simulink model "TestBenchModel"  (R2019b)
settings: Solver=VariableStepAuto  StartTime=0.0  StopTime=60  FixedStep=0.0001  RelTol=1e-3  EnableMultiTasking=on
InitFcn:
  | TestBenchData;
StartFcn:
  | TestBenchData;
values from neighbouring files (symbols this model uses):
  C = 0.0056    [TestBenchData.m]
  C1 = C    (= 0.0056)    [TestBenchData.m]
  C2 = C1    (= 0.0056)    [TestBenchData.m]
  C3 = C1    (= 0.0056)    [TestBenchData.m]
  C4 = C1    (= 0.0056)    [TestBenchData.m]
  C5 = C1    (= 0.0056)    [TestBenchData.m]
  C6 = C1    (= 0.0056)    [TestBenchData.m]
  Cfc = 0.35    [TestBenchData.m]
  Fs = 1000    [TestBenchData.m]
  glg = 4    [TestBenchData.m]
  gug = 3    [TestBenchData.m]
  Ic1 = 0.05*10^(-3)    (= 5e-05)    [TestBenchData.m]
  Ic4 = Ic3    (= 0.00012)    [TestBenchData.m]
  Ic_mf = 1.1420e-04    (= 0.0001142)    [TestBenchData.m]
  Ifc_1 = 0.003*10^(-3)    (= 3e-06)    [TestBenchData.m]
  Ifc_2 = 0.003*10^(-3)    (= 3e-06)    [TestBenchData.m]
  Imotor = 0.00068    [TestBenchData.m]
  Iprop = gml^2*I_ML + I_GL + Iprop0    [TestBenchData.m]
  Kc1 = 41.9*10^3    (= 41900)    [TestBenchData.m]
  Kc2 = Kc1    (= 41900)    [TestBenchData.m]
  Kc3 = 31*10^3    (= 31000)    [TestBenchData.m]
  Kc4 = Kc3    (= 31000)    [TestBenchData.m]
  Kc5 = 138*10^3    (= 138000)    [TestBenchData.m]
  Kc6 = Kc5    (= 138000)    [TestBenchData.m]
  Kc_mf = 1.9039e+05    (= 190390)    [TestBenchData.m]
  Kfc = 90    [TestBenchData.m]
  Klg = 44.3*10^3    (= 44300)    [TestBenchData.m]
  Km1 = 5.4*10^3    (= 5400)    [TestBenchData.m]
  Km2 = 20*10^3    (= 20000)    [TestBenchData.m]
  Kug = 43.3*10^3    (= 43300)    [TestBenchData.m]
  lg = C1    (= 0.0056)    [TestBenchData.m]
  M1 = S1    (= 0.0056)    [TestBenchData.m]
  M2 = M1    (= 0.0056)    [TestBenchData.m]
  n = 3221    [TestBenchData.m]
  n_idle = 0    [TestBenchData.m]
  Nmill = 12    [TestBenchData.m]
  P = 1150    [TestBenchData.m]
  prop_blades = 4    [TestBenchData.m]
  S = 0.0056    [TestBenchData.m]
  S1 = S    (= 0.0056)    [TestBenchData.m]
  S2 = S1    (= 0.0056)    [TestBenchData.m]
  S3 = S1    (= 0.0056)    [TestBenchData.m]
  S4 = S1    (= 0.0056)    [TestBenchData.m]
  S5 = S1    (= 0.0056)    [TestBenchData.m]
  T = P/(n/9.55)    (= 3.40965538653)    [TestBenchData.m]
  Tice = 100000    [TestBenchData.m]
  To = 0.2    [TestBenchData.m]
  Todelta = 0.5    [TestBenchData.m]
  ug = C1    (= 0.0056)    [TestBenchData.m]
  W = 131.9469    [TestBenchData.m]
  x4 = 0.06/4    (= 0.015)    [TestBenchData.m]
  x8 = 0.02/4    (= 0.005)    [TestBenchData.m]
  Z = 4    [TestBenchData.m]
  z1 = 17    [TestBenchData.m]
  z2 = 42    [TestBenchData.m]
undefined symbols (not defined in the file or in its folder): C1_22, C1_3, C_crank, C_cyl, Data, Iem, Is1, Is2, Is3, Is4, Is5, K1_11, K1_13, K1_15, K1_21, K1_23, K1_5, K1_7, K1_9, Ks1, Ks2, Ks3, Ks4, Ks5, Ks_mf, RPM, Tu
libraries: fl_lib x201, nesl_utility x92, simulink x22, dspstat3 x1
(part 2 of 3)

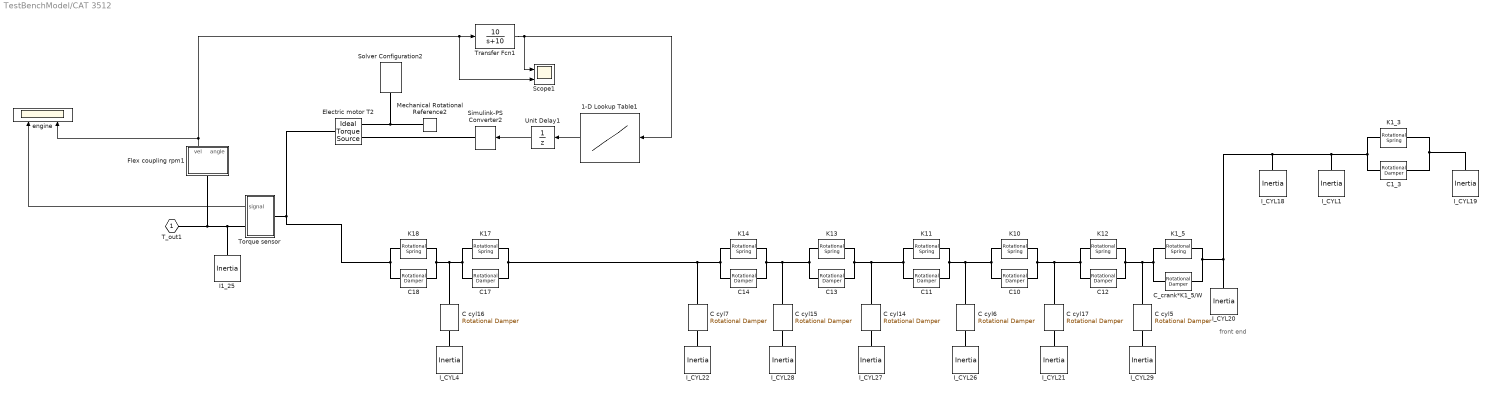
== system TestBenchModel/CAT 3512 ==
  note: front end
  " K1_5" : fl_lib/Mechanical/Rotational Elements/Rotational Spring  spr_rate=K1_5 N*m/rad  w_specify=off  w_priority=None  w=0 rad/s  w_nominal_specify=off  w_nominal_unit=rad/s  w_nominal_value=1  t_specify=off  t_priority=None  t=0 N*m  t_nominal_specify=off  t_nominal_unit=N*m  t_nominal_value=1  phi_specify=on  phi_priority=High  phi=0 rad  phi_nominal_specify=off  phi_nominal_unit=rad  phi_nominal_value=1
      settings: SourceProductName=Simscape
  " engine" : Scope  NumInputPorts=2
  1-D Lookup Table1 : Lookup_n-D  NumberOfTableDimensions=1  BreakpointsForDimension1=RPM  Table=Tu  RndMeth=Simplest  InputSameDT=on
  C cyl{5..7,14..15,17} (6 alike) : fl_lib/Mechanical/Rotational Elements/Rotational Damper  D=C_cyl N*m/(rad/s)  w_specify=off  w_priority=None  w=0 rad/s  w_nominal_specify=off  w_nominal_unit=rad/s  w_nominal_value=1  t_specify=off  t_priority=None  t=0 N*m  t_nominal_specify=off  t_nominal_unit=N*m  t_nominal_value=1
  C cyl16 : fl_lib/Mechanical/Rotational Elements/Rotational Damper  D=C1_22 N*m/(rad/s)  w_specify=off  w_priority=None  w=0 rad/s  w_nominal_specify=off  w_nominal_unit=rad/s  w_nominal_value=1  t_specify=off  t_priority=None  t=0 N*m  t_nominal_specify=off  t_nominal_unit=N*m  t_nominal_value=1
  C10 : fl_lib/Mechanical/Rotational Elements/Rotational Damper  D=C_crank*K1_9/W N*m/(rad/s)  w_specify=off  w_priority=None  w=0 rad/s  w_nominal_specify=off  w_nominal_unit=rad/s  w_nominal_value=1  t_specify=off  t_priority=None  t=0 N*m  t_nominal_specify=off  t_nominal_unit=N*m  t_nominal_value=1
      settings: AttributesFormatString=%<D>
  C11 : fl_lib/Mechanical/Rotational Elements/Rotational Damper  D=C_crank*K1_11/W N*m/(rad/s)  w_specify=off  w_priority=None  w=0 rad/s  w_nominal_specify=off  w_nominal_unit=rad/s  w_nominal_value=1  t_specify=off  t_priority=None  t=0 N*m  t_nominal_specify=off  t_nominal_unit=N*m  t_nominal_value=1
      settings: AttributesFormatString=%<D>
  C12 : fl_lib/Mechanical/Rotational Elements/Rotational Damper  D=C_crank*K1_7/W N*m/(rad/s)  w_specify=off  w_priority=None  w=0 rad/s  w_nominal_specify=off  w_nominal_unit=rad/s  w_nominal_value=1  t_specify=off  t_priority=None  t=0 N*m  t_nominal_specify=off  t_nominal_unit=N*m  t_nominal_value=1
      settings: AttributesFormatString=%<D>
  C13 : fl_lib/Mechanical/Rotational Elements/Rotational Damper  D=C_crank*K1_13/W N*m/(rad/s)  w_specify=off  w_priority=None  w=0 rad/s  w_nominal_specify=off  w_nominal_unit=rad/s  w_nominal_value=1  t_specify=off  t_priority=None  t=0 N*m  t_nominal_specify=off  t_nominal_unit=N*m  t_nominal_value=1
      settings: AttributesFormatString=%<D>
  C14 : fl_lib/Mechanical/Rotational Elements/Rotational Damper  D=C_crank*K1_15/W N*m/(rad/s)  w_specify=off  w_priority=None  w=0 rad/s  w_nominal_specify=off  w_nominal_unit=rad/s  w_nominal_value=1  t_specify=off  t_priority=None  t=0 N*m  t_nominal_specify=off  t_nominal_unit=N*m  t_nominal_value=1
      settings: AttributesFormatString=%<D>
  C17 : fl_lib/Mechanical/Rotational Elements/Rotational Damper  D=C_crank*K1_21/W N*m/(rad/s)  w_specify=off  w_priority=None  w=0 rad/s  w_nominal_specify=off  w_nominal_unit=rad/s  w_nominal_value=1  t_specify=off  t_priority=None  t=0 N*m  t_nominal_specify=off  t_nominal_unit=N*m  t_nominal_value=1
      settings: AttributesFormatString=%<D>
  C18 : fl_lib/Mechanical/Rotational Elements/Rotational Damper  D=C_crank*K1_23/W N*m/(rad/s)  w_specify=off  w_priority=None  w=0 rad/s  w_nominal_specify=off  w_nominal_unit=rad/s  w_nominal_value=1  t_specify=off  t_priority=None  t=0 N*m  t_nominal_specify=off  t_nominal_unit=N*m  t_nominal_value=1
      settings: AttributesFormatString=%<D>
  "C1_3 " : fl_lib/Mechanical/Rotational Elements/Rotational Damper  D=C1_3 N*m/(rad/s)  w_specify=off  w_priority=None  w=0 rad/s  w_nominal_specify=off  w_nominal_unit=rad/s  w_nominal_value=1  t_specify=off  t_priority=None  t=0 N*m  t_nominal_specify=off  t_nominal_unit=N*m  t_nominal_value=1
  C_crank*K1_5/W : fl_lib/Mechanical/Rotational Elements/Rotational Damper  D=C_crank*K1_5/W N*m/(rad/s)  w_specify=off  w_priority=None  w=0 rad/s  w_nominal_specify=off  w_nominal_unit=rad/s  w_nominal_value=1  t_specify=off  t_priority=None  t=0 N*m  t_nominal_specify=off  t_nominal_unit=N*m  t_nominal_value=1
  Electric motor T2 : fl_lib/Mechanical/Mechanical Sources/Ideal Torque Source
  Flex coupling rpm1 : Subsystem
  I1_25 : fl_lib/Mechanical/Rotational Elements/Inertia  inertia=I1_25 kg*m^2  w_specify=on  w_priority=High  w=n_idle rpm  w_nominal_specify=off  w_nominal_unit=rad/s  w_nominal_value=1  t_specify=off  t_priority=None  t=0 N*m  t_nominal_specify=off  t_nominal_unit=N*m  t_nominal_value=1
  I_CYL1 : fl_lib/Mechanical/Rotational Elements/Inertia  inertia=I1_3hsg kg*m^2  w_specify=on  w_priority=High  w=n_idle rpm  w_nominal_specify=off  w_nominal_unit=rad/s  w_nominal_value=1  t_specify=off  t_priority=None  t=0 N*m  t_nominal_specify=off  t_nominal_unit=N*m  t_nominal_value=1
      settings: AttributesFormatString=%<inertia>
  I_CYL18 : fl_lib/Mechanical/Rotational Elements/Inertia  inertia=I1_3adap kg*m^2  w_specify=on  w_priority=High  w=n_idle rpm  w_nominal_specify=off  w_nominal_unit=rad/s  w_nominal_value=1  t_specify=off  t_priority=None  t=0 N*m  t_nominal_specify=off  t_nominal_unit=N*m  t_nominal_value=1
      settings: AttributesFormatString=%<inertia>
  I_CYL19 : fl_lib/Mechanical/Rotational Elements/Inertia  inertia=I1_3ring kg*m^2  w_specify=on  w_priority=High  w=n_idle rpm  w_nominal_specify=off  w_nominal_unit=rad/s  w_nominal_value=1  t_specify=off  t_priority=None  t=0 N*m  t_nominal_specify=off  t_nominal_unit=N*m  t_nominal_value=1
      settings: AttributesFormatString=%<inertia>
  I_CYL20 : fl_lib/Mechanical/Rotational Elements/Inertia  inertia=I1_4 kg*m^2  w_specify=on  w_priority=High  w=n_idle rpm  w_nominal_specify=off  w_nominal_unit=rad/s  w_nominal_value=1  t_specify=off  t_priority=None  t=0 N*m  t_nominal_specify=off  t_nominal_unit=N*m  t_nominal_value=1
      settings: AttributesFormatString=%<inertia>
  I_CYL21 : fl_lib/Mechanical/Rotational Elements/Inertia  inertia=I1_8 kg*m^2  w_specify=on  w_priority=High  w=n_idle rpm  w_nominal_specify=off  w_nominal_unit=rad/s  w_nominal_value=1  t_specify=off  t_priority=None  t=0 N*m  t_nominal_specify=off  t_nominal_unit=N*m  t_nominal_value=1
      settings: AttributesFormatString=%<inertia>
  I_CYL22 : fl_lib/Mechanical/Rotational Elements/Inertia  inertia=I1_16 kg*m^2  w_specify=on  w_priority=High  w=n_idle rpm  w_nominal_specify=off  w_nominal_unit=rad/s  w_nominal_value=1  t_specify=off  t_priority=None  t=0 N*m  t_nominal_specify=off  t_nominal_unit=N*m  t_nominal_value=1
      settings: AttributesFormatString=%<inertia>
  I_CYL26 : fl_lib/Mechanical/Rotational Elements/Inertia  inertia=I1_10 kg*m^2  w_specify=on  w_priority=High  w=n_idle rpm  w_nominal_specify=off  w_nominal_unit=rad/s  w_nominal_value=1  t_specify=off  t_priority=None  t=0 N*m  t_nominal_specify=off  t_nominal_unit=N*m  t_nominal_value=1
      settings: AttributesFormatString=%<inertia>
  I_CYL27 : fl_lib/Mechanical/Rotational Elements/Inertia  inertia=I1_12 kg*m^2  w_specify=on  w_priority=High  w=n_idle rpm  w_nominal_specify=off  w_nominal_unit=rad/s  w_nominal_value=1  t_specify=off  t_priority=None  t=0 N*m  t_nominal_specify=off  t_nominal_unit=N*m  t_nominal_value=1
      settings: AttributesFormatString=%<inertia>
  I_CYL28 : fl_lib/Mechanical/Rotational Elements/Inertia  inertia=I1_14 kg*m^2  w_specify=on  w_priority=High  w=n_idle rpm  w_nominal_specify=off  w_nominal_unit=rad/s  w_nominal_value=1  t_specify=off  t_priority=None  t=0 N*m  t_nominal_specify=off  t_nominal_unit=N*m  t_nominal_value=1
      settings: AttributesFormatString=%<inertia>
  I_CYL29 : fl_lib/Mechanical/Rotational Elements/Inertia  inertia=I1_6 kg*m^2  w_specify=on  w_priority=High  w=n_idle rpm  w_nominal_specify=off  w_nominal_unit=rad/s  w_nominal_value=1  t_specify=off  t_priority=None  t=0 N*m  t_nominal_specify=off  t_nominal_unit=N*m  t_nominal_value=1
      settings: AttributesFormatString=%<inertia>
  I_CYL4 : fl_lib/Mechanical/Rotational Elements/Inertia  inertia=I1_22 kg*m^2  w_specify=on  w_priority=High  w=n_idle rpm  w_nominal_specify=off  w_nominal_unit=rad/s  w_nominal_value=1  t_specify=off  t_priority=None  t=0 N*m  t_nominal_specify=off  t_nominal_unit=N*m  t_nominal_value=1
      settings: AttributesFormatString=%<inertia>
  K10 : fl_lib/Mechanical/Rotational Elements/Rotational Spring  spr_rate=K1_9 N*m/rad  w_specify=off  w_priority=None  w=0 rad/s  w_nominal_specify=off  w_nominal_unit=rad/s  w_nominal_value=1  t_specify=off  t_priority=None  t=0 N*m  t_nominal_specify=off  t_nominal_unit=N*m  t_nominal_value=1  phi_specify=on  phi_priority=High  phi=0 rad  phi_nominal_specify=off  phi_nominal_unit=rad  phi_nominal_value=1
      settings: AttributesFormatString=%<spr_rate>  SourceProductName=Simscape
  K11 : fl_lib/Mechanical/Rotational Elements/Rotational Spring  spr_rate=K1_11 N*m/rad  w_specify=off  w_priority=None  w=0 rad/s  w_nominal_specify=off  w_nominal_unit=rad/s  w_nominal_value=1  t_specify=off  t_priority=None  t=0 N*m  t_nominal_specify=off  t_nominal_unit=N*m  t_nominal_value=1  phi_specify=on  phi_priority=High  phi=0 rad  phi_nominal_specify=off  phi_nominal_unit=rad  phi_nominal_value=1
      settings: AttributesFormatString=%<spr_rate>  SourceProductName=Simscape
  K12 : fl_lib/Mechanical/Rotational Elements/Rotational Spring  spr_rate=K1_7 N*m/rad  w_specify=off  w_priority=None  w=0 rad/s  w_nominal_specify=off  w_nominal_unit=rad/s  w_nominal_value=1  t_specify=off  t_priority=None  t=0 N*m  t_nominal_specify=off  t_nominal_unit=N*m  t_nominal_value=1  phi_specify=on  phi_priority=High  phi=0 rad  phi_nominal_specify=off  phi_nominal_unit=rad  phi_nominal_value=1
      settings: AttributesFormatString=%<spr_rate>  SourceProductName=Simscape
  K13 : fl_lib/Mechanical/Rotational Elements/Rotational Spring  spr_rate=K1_13 N*m/rad  w_specify=off  w_priority=None  w=0 rad/s  w_nominal_specify=off  w_nominal_unit=rad/s  w_nominal_value=1  t_specify=off  t_priority=None  t=0 N*m  t_nominal_specify=off  t_nominal_unit=N*m  t_nominal_value=1  phi_specify=on  phi_priority=High  phi=0 rad  phi_nominal_specify=off  phi_nominal_unit=rad  phi_nominal_value=1
      settings: AttributesFormatString=%<spr_rate>  SourceProductName=Simscape
  K14 : fl_lib/Mechanical/Rotational Elements/Rotational Spring  spr_rate=K1_15 N*m/rad  w_specify=off  w_priority=None  w=0 rad/s  w_nominal_specify=off  w_nominal_unit=rad/s  w_nominal_value=1  t_specify=off  t_priority=None  t=0 N*m  t_nominal_specify=off  t_nominal_unit=N*m  t_nominal_value=1  phi_specify=on  phi_priority=High  phi=0 rad  phi_nominal_specify=off  phi_nominal_unit=rad  phi_nominal_value=1
      settings: AttributesFormatString=%<spr_rate>  SourceProductName=Simscape
  K17 : fl_lib/Mechanical/Rotational Elements/Rotational Spring  spr_rate=K1_21 N*m/rad  w_specify=off  w_priority=None  w=0 rad/s  w_nominal_specify=off  w_nominal_unit=rad/s  w_nominal_value=1  t_specify=off  t_priority=None  t=0 N*m  t_nominal_specify=off  t_nominal_unit=N*m  t_nominal_value=1  phi_specify=on  phi_priority=High  phi=0 rad  phi_nominal_specify=off  phi_nominal_unit=rad  phi_nominal_value=1
      settings: AttributesFormatString=%<spr_rate>  SourceProductName=Simscape
  K18 : fl_lib/Mechanical/Rotational Elements/Rotational Spring  spr_rate=K1_23 N*m/rad  w_specify=off  w_priority=None  w=0 rad/s  w_nominal_specify=off  w_nominal_unit=rad/s  w_nominal_value=1  t_specify=off  t_priority=None  t=0 N*m  t_nominal_specify=off  t_nominal_unit=N*m  t_nominal_value=1  phi_specify=on  phi_priority=High  phi=0 rad  phi_nominal_specify=off  phi_nominal_unit=rad  phi_nominal_value=1
      settings: AttributesFormatString=%<spr_rate>  SourceProductName=Simscape
  K1_3 : fl_lib/Mechanical/Rotational Elements/Rotational Spring  spr_rate=K1_3 N*m/rad  w_specify=off  w_priority=None  w=0 rad/s  w_nominal_specify=off  w_nominal_unit=rad/s  w_nominal_value=1  t_specify=off  t_priority=None  t=0 N*m  t_nominal_specify=off  t_nominal_unit=N*m  t_nominal_value=1  phi_specify=on  phi_priority=High  phi=0 rad  phi_nominal_specify=off  phi_nominal_unit=rad  phi_nominal_value=1
      settings: SourceProductName=Simscape
  Mechanical Rotational Reference2 : fl_lib/Mechanical/Rotational Elements/Mechanical Rotational Reference
  Scope1 : Scope  NumInputPorts=2
  Simulink-PS Converter2 : nesl_utility/Simulink-PS Converter  PhysicalDomain=network_engine_domain  SubClassName=ps_input  LeftPortType=input  RightPortType=output  PseudoPeriodic=off  Frequencies=[]  NoiseDistribution=none  NoiseParameters=[]  Unit=N*m  AffineConversion=off  FilteringAndDerivatives=zero  SimscapeFilterOrder=1  InputFilterTimeConstant=.001  UdotUserProvided=0
  Solver Configuration2 : nesl_utility/Solver Configuration  PhysicalDomain=network_engine_domain  SubClassName=solver  LeftPortType=input  RightPortType=generic  Tones=[]  Harmonics=[]  SimulateNoise=off  Profile=off  UseLocalSampling=off  EnableSwitchedLinearOptims=on  FrequencyDomain=off  UseCCode=off  RelTol=0.001  AbsTol=1e-06  MinStep=1e-09  ToWorkspace=off  RevertToSquareIcSolve=off  NumHomotopyIterations=100  PhasorMode=off  PhasorModeNumHarmonics=1  DoDC=off  ResidualTolerance=1e-9  UseLocalSolver=off  LocalSolverChoice=NE_BACKWARD_EULER_ADVANCER  LocalSolverSampleTime=.001  DoFixedCost=off  MaxNonlinIter=3  MaxModeIter=2  LinearAlgebra=Sparse  EquationFormulation=NE_TIME_EF  DelaysMemoryBudget=1024  AutomaticFiltering=on  FilteringTimeConstant=0.001  PartitionStorageMethod=AS_NEEDED  PartitionMemoryBudget=1024  PartitionMethod=FAST
  Torque sensor : Subsystem
  Transfer Fcn1 : TransferFcn  Numerator=[10]  Denominator=[1 10]
  Unit Delay1 : UnitDelay  SampleTime=-1  HasFrameUpgradeWarning=on
  T_out1 : PMIOPort  Side=Left
  wires:
  Flex coupling rpm1/1(vel) -> Transfer Fcn1/1, Scope1/2, " engine"/2
  Transfer Fcn1/1 -> 1-D Lookup Table1/1, Scope1/1
  1-D Lookup Table1/1 -> Unit Delay1/1
  Unit Delay1/1 -> Simulink-PS Converter2/1
  Torque sensor/1(signal) -> " engine"/1
  connections:
  Flex coupling rpm1/LConn1 -- T_out1/RConn1 -- Torque sensor/RConn1 -- I1_25/LConn1
  Solver Configuration2/RConn1 -- Electric motor T2/RConn2 -- Mechanical Rotational Reference2/LConn1
  K18/RConn1 -- Electric motor T2/LConn1 -- Torque sensor/LConn1 -- C18/RConn1
  Simulink-PS Converter2/RConn1 -- Electric motor T2/RConn1
  K1_3/LConn1 -- "C1_3 "/LConn1 -- I_CYL19/LConn1
  "C1_3 "/RConn1 -- I_CYL18/LConn1 -- I_CYL20/LConn1 -- C_crank*K1_5/W/LConn1 -- " K1_5"/LConn1 -- I_CYL1/LConn1 -- K1_3/RConn1
  C12/LConn1 -- K12/LConn1 -- C cyl5/RConn1 -- C_crank*K1_5/W/RConn1 -- " K1_5"/RConn1
  C10/LConn1 -- K10/LConn1 -- K12/RConn1 -- C12/RConn1 -- C cyl17/RConn1
  C11/LConn1 -- K11/LConn1 -- K10/RConn1 -- C10/RConn1 -- C cyl6/RConn1
  K11/RConn1 -- C11/RConn1 -- C cyl14/RConn1 -- C13/LConn1 -- K13/LConn1
  C14/LConn1 -- K14/LConn1 -- K13/RConn1 -- C13/RConn1 -- C cyl15/RConn1
  K17/LConn1 -- C17/LConn1 -- C cyl7/RConn1 -- K14/RConn1 -- C14/RConn1
  K17/RConn1 -- C17/RConn1 -- C cyl16/RConn1 -- K18/LConn1 -- C18/LConn1
  I_CYL21/LConn1 -- C cyl17/LConn1
  I_CYL28/LConn1 -- C cyl15/LConn1
  I_CYL22/LConn1 -- C cyl7/LConn1
  I_CYL4/LConn1 -- C cyl16/LConn1
  I_CYL26/LConn1 -- C cyl6/LConn1
  I_CYL27/LConn1 -- C cyl14/LConn1
  I_CYL29/LConn1 -- C cyl5/LConn1

== system TestBenchModel/Flex coupling rpm ==
  Constant : Constant  Value=9.55
  Ideal Rotational Motion Sensor1 : fl_lib/Mechanical/Mechanical Sensors/Ideal Rotational Motion Sensor  offset=0 rad
  Mechanical Rotational Reference3 : fl_lib/Mechanical/Rotational Elements/Mechanical Rotational Reference
  PS-Simulink Converter1 : nesl_utility/PS-Simulink Converter  PhysicalDomain=network_engine_domain  SubClassName=ps_output  LeftPortType=input  RightPortType=output  PseudoPeriodic=off  Frequencies=[]  Unit=1  AffineConversion=off
  PS-Simulink Converter2 : nesl_utility/PS-Simulink Converter  PhysicalDomain=network_engine_domain  SubClassName=ps_output  LeftPortType=input  RightPortType=output  PseudoPeriodic=off  Frequencies=[]  Unit=1  AffineConversion=off
  Product : Product  RndMeth=Zero
  Scope : Scope
  in : PMIOPort  Side=Left
  vel : Outport
  angle : Outport  Port=2
  wires:
  PS-Simulink Converter1/1 -> angle/1
  PS-Simulink Converter2/1 -> Scope/1, Product/2
  Constant/1 -> Product/1
  Product/1 -> vel/1
  connections:
  Mechanical Rotational Reference3/LConn1 -- Ideal Rotational Motion Sensor1/RConn1
  PS-Simulink Converter2/LConn1 -- Ideal Rotational Motion Sensor1/RConn2
  in/RConn1 -- Ideal Rotational Motion Sensor1/LConn1
  PS-Simulink Converter1/LConn1 -- Ideal Rotational Motion Sensor1/RConn3

== system TestBenchModel/Gear mesh torque ==
  Ideal Torque Sensor1 : fl_lib/Mechanical/Mechanical Sensors/Ideal Torque Sensor
  PS-Simulink Converter : nesl_utility/PS-Simulink Converter  PhysicalDomain=network_engine_domain  SubClassName=ps_output  LeftPortType=input  RightPortType=output  PseudoPeriodic=off  Frequencies=[]  Unit=N*m  AffineConversion=off
  T_in : PMIOPort  Side=Left
  T_out : PMIOPort  Port=2  Side=Right
  signal : Outport
  wires:
  PS-Simulink Converter/1 -> signal/1
  connections:
  PS-Simulink Converter/LConn1 -- Ideal Torque Sensor1/RConn2
  T_in/RConn1 -- Ideal Torque Sensor1/LConn1
  T_out/RConn1 -- Ideal Torque Sensor1/RConn1

== system TestBenchModel/Prop shaft rpm ==
  Constant : Constant  Value=9.55
  Ideal Rotational Motion Sensor1 : fl_lib/Mechanical/Mechanical Sensors/Ideal Rotational Motion Sensor  offset=0 rad
  Mechanical Rotational Reference3 : fl_lib/Mechanical/Rotational Elements/Mechanical Rotational Reference
  PS-Simulink Converter1 : nesl_utility/PS-Simulink Converter  PhysicalDomain=network_engine_domain  SubClassName=ps_output  LeftPortType=input  RightPortType=output  PseudoPeriodic=off  Frequencies=[]  Unit=1  AffineConversion=off
  PS-Simulink Converter2 : nesl_utility/PS-Simulink Converter  PhysicalDomain=network_engine_domain  SubClassName=ps_output  LeftPortType=input  RightPortType=output  PseudoPeriodic=off  Frequencies=[]  Unit=1  AffineConversion=off
  Product : Product  RndMeth=Zero
  in : PMIOPort  Side=Left
  vel : Outport
  angle : Outport  Port=2
  wires:
  PS-Simulink Converter1/1 -> angle/1
  PS-Simulink Converter2/1 -> Product/2
  Constant/1 -> Product/1
  Product/1 -> vel/1
  connections:
  Mechanical Rotational Reference3/LConn1 -- Ideal Rotational Motion Sensor1/RConn1
  PS-Simulink Converter2/LConn1 -- Ideal Rotational Motion Sensor1/RConn2
  in/RConn1 -- Ideal Rotational Motion Sensor1/LConn1
  PS-Simulink Converter1/LConn1 -- Ideal Rotational Motion Sensor1/RConn3

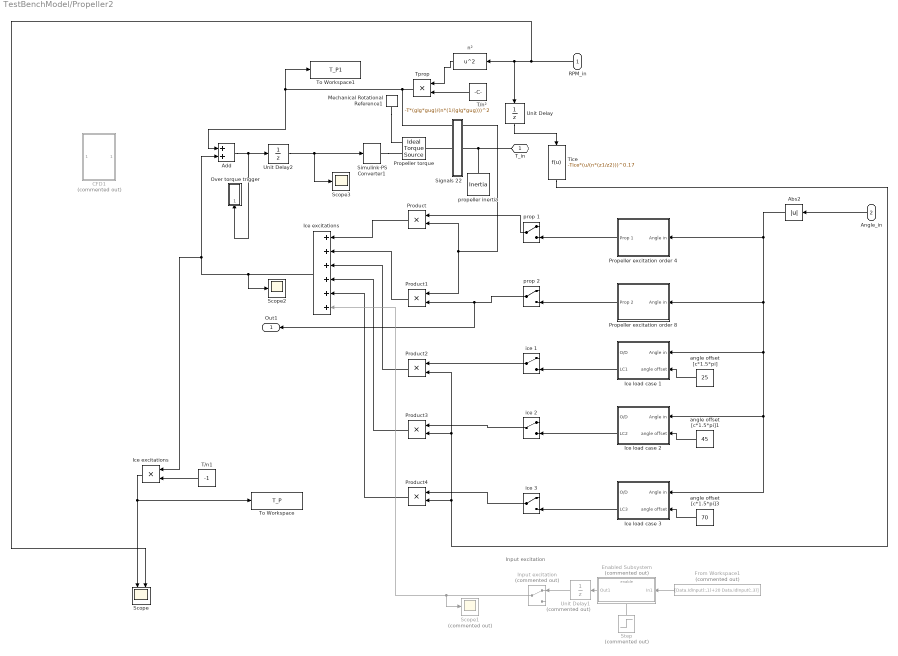
== system TestBenchModel/Propeller2 ==
  note: Input excitation
  RPM_in : Inport
  Angle_in : Inport  Port=2
  " Ice excitations" : Product  RndMeth=Zero
  " ice 1" : ManualSwitch
  " ice 2" : ManualSwitch
  " ice 3" : ManualSwitch
  " prop 1" : ManualSwitch
  Abs2 : Abs
  Add : Sum
  CFD1 : Subsystem  Commented=on
  Enabled Subsystem : Subsystem  Commented=on  TreatAsAtomicUnit=on
  From Workspace1 : FromWorkspace  Commented=on  VariableName=[Data.IdInput(:,1)+20 Data.IdInput(:,3)]  SampleTime=0  OutputAfterFinalValue=Setting to zero
  Ice excitations : Sum  Inputs=++++++
  Ice load case 1 : Subsystem
  Ice load case 2 : Subsystem
  Ice load case 3 : Subsystem
  Input excitation : ManualSwitch  Commented=on
  Mechanical Rotational Reference1 : fl_lib/Mechanical/Rotational Elements/Mechanical Rotational Reference
  Over torque trigger : Subsystem
  Product{,1..4} (5 alike) : Product  RndMeth=Zero
  Propeller excitation order 4 : Subsystem
  Propeller excitation order 8 : Subsystem
  Propeller torque : fl_lib/Mechanical/Mechanical Sources/Ideal Torque Source
  Scope : Scope  NumInputPorts=2
  Scope1 : Scope  Commented=on
  Scope2 : Scope
  Scope3 : Scope
  "Signals 22 " : Subsystem
  Simulink-PS Converter1 : nesl_utility/Simulink-PS Converter  PhysicalDomain=network_engine_domain  SubClassName=ps_input  LeftPortType=input  RightPortType=output  PseudoPeriodic=off  Frequencies=[]  NoiseDistribution=none  NoiseParameters=[]  Unit=N*m  AffineConversion=off  FilteringAndDerivatives=zero  SimscapeFilterOrder=1  InputFilterTimeConstant=.001  UdotUserProvided=0
  Step : Step  Commented=on  Time=20  SampleTime=0
  T/n1 : Constant  Value=-1
  T/n² : Constant  Value=-T*(glg*gug)/(n*(1/(glg*gug)))^2
  Tice : Fcn  Expr=-Tice*(u/(n*(z1/z2)))^0.17
  To Workspace : ToWorkspace  VariableName=T_P  SaveFormat=Timeseries  SampleTime=-1
  To Workspace1 : ToWorkspace  VariableName=T_P1  SaveFormat=Timeseries  SampleTime=-1
  Tprop : Product  RndMeth=Zero
  Unit Delay : UnitDelay  SampleTime=-1  HasFrameUpgradeWarning=on
  Unit Delay1 : UnitDelay  Commented=on  SampleTime=-1  HasFrameUpgradeWarning=on
  Unit Delay2 : UnitDelay  SampleTime=-1  HasFrameUpgradeWarning=on
  angle offset [c*1.5*pi] : Constant  Value=25
  angle offset [c*1.5*pi]1 : Constant  Value=45
  angle offset [c*1.5*pi]3 : Constant  Value=70
  n² : Fcn  Expr=u^2
  prop 2 : ManualSwitch
  propeller inertia : fl_lib/Mechanical/Rotational Elements/Inertia  inertia=Iprop+Is5/2 kg*m^2  w_specify=on  w_priority=High  w=0 rpm  w_nominal_specify=off  w_nominal_unit=rad/s  w_nominal_value=1  t_specify=off  t_priority=None  t=0 N*m  t_nominal_specify=off  t_nominal_unit=N*m  t_nominal_value=1
  T_in : PMIOPort  Side=Left
  Out1 : Outport
  wires:
  T/n²/1 -> Tprop/2
  n²/1 -> Tprop/1
  RPM_in/1 -> Scope/2, n²/1, Unit Delay/1
  Angle_in/1 -> Abs2/1
  Product/1 -> Ice excitations/1
  Product1/1 -> Ice excitations/2
  Propeller excitation order 8/1(Prop 2) -> prop 2/2
  Product2/1 -> Ice excitations/3
  Tprop/1 -> Product1/1, Product/2, Add/1, To Workspace1/1
  Unit Delay/1 -> Tice/1
  Propeller excitation order 4/1(Prop 1) -> " prop 1"/2
  Unit Delay2/1 -> Scope3/1, Simulink-PS Converter1/1
  " ice 1"/1 -> Product2/1
  " prop 1"/1 -> Product/1
  prop 2/1 -> Out1/1, Product1/2
  Abs2/1 -> Propeller excitation order 4/1(Angle in), Ice load case 3/1(Angle in), Ice load case 2/1(Angle in), Ice load case 1/1(Angle in), Propeller excitation order 8/1(Angle in)
  angle offset [c*1.5*pi]1/1 -> Ice load case 2/2(angle offset)
  angle offset [c*1.5*pi]3/1 -> Ice load case 3/2(angle offset)
  angle offset [c*1.5*pi]/1 -> Ice load case 1/2(angle offset)
  Ice load case 1/2(LC1) -> " ice 1"/2
  Tice/1 -> Product4/2, Product3/2, Product2/2
  Product4/1 -> Ice excitations/5
  Product3/1 -> Ice excitations/4
  Ice load case 2/2(LC2) -> " ice 2"/2
  " ice 2"/1 -> Product3/1
  Ice load case 3/2(LC3) -> " ice 3"/2
  " ice 3"/1 -> Product4/1
  T/n1/1 -> " Ice excitations"/2
  " Ice excitations"/1 -> To Workspace/1, Scope/1
  Ice excitations/1 -> Scope2/1, " Ice excitations"/1, Add/2
  Add/1 -> Unit Delay2/1, Over torque trigger/1(O/D in)
  Input excitation/1 -> Scope1/1, Ice excitations/6
  Step/1 -> Enabled Subsystem/Enable
  From Workspace1/1 -> Enabled Subsystem/1(In1)
  Enabled Subsystem/1(Out1) -> Unit Delay1/1
  Unit Delay1/1 -> Input excitation/1
  connections:
  Mechanical Rotational Reference1/LConn1 -- Propeller torque/RConn2
  Simulink-PS Converter1/RConn1 -- Propeller torque/RConn1
  T_in/RConn1 -- "Signals 22 "/LConn1 -- propeller inertia/LConn1
  "Signals 22 "/RConn1 -- Propeller torque/LConn1

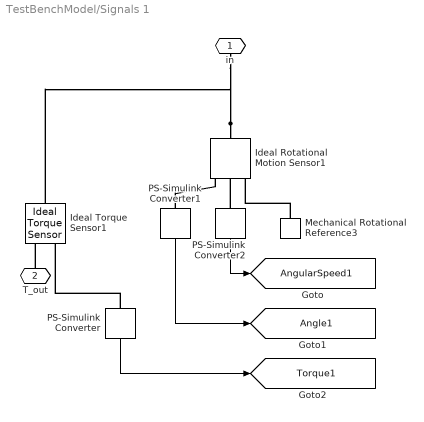
== system TestBenchModel/Signals 1 ==
  Ideal Rotational Motion Sensor1 : fl_lib/Mechanical/Mechanical Sensors/Ideal Rotational Motion Sensor  offset=0 rad
  Ideal Torque Sensor1 : fl_lib/Mechanical/Mechanical Sensors/Ideal Torque Sensor
  Mechanical Rotational Reference3 : fl_lib/Mechanical/Rotational Elements/Mechanical Rotational Reference
  PS-Simulink Converter : nesl_utility/PS-Simulink Converter  PhysicalDomain=network_engine_domain  SubClassName=ps_output  LeftPortType=input  RightPortType=output  PseudoPeriodic=off  Frequencies=[]  Unit=N*m  AffineConversion=off
  PS-Simulink Converter1 : nesl_utility/PS-Simulink Converter  PhysicalDomain=network_engine_domain  SubClassName=ps_output  LeftPortType=input  RightPortType=output  PseudoPeriodic=off  Frequencies=[]  Unit=1  AffineConversion=off
  PS-Simulink Converter2 : nesl_utility/PS-Simulink Converter  PhysicalDomain=network_engine_domain  SubClassName=ps_output  LeftPortType=input  RightPortType=output  PseudoPeriodic=off  Frequencies=[]  Unit=1  AffineConversion=off
  in : PMIOPort  Side=Left
  T_out : PMIOPort  Port=2  Side=Right
  tag scope: Angle1=global, AngularSpeed1=global, Torque1=global
  wires:
  PS-Simulink Converter/1 -> [Torque1]
  PS-Simulink Converter1/1 -> [Angle1]
  PS-Simulink Converter2/1 -> [AngularSpeed1]
  connections:
  PS-Simulink Converter/LConn1 -- Ideal Torque Sensor1/RConn2
  T_out/RConn1 -- Ideal Torque Sensor1/RConn1
  Mechanical Rotational Reference3/LConn1 -- Ideal Rotational Motion Sensor1/RConn1
  PS-Simulink Converter2/LConn1 -- Ideal Rotational Motion Sensor1/RConn2
  Ideal Rotational Motion Sensor1/LConn1 -- Ideal Torque Sensor1/LConn1 -- in/RConn1
  PS-Simulink Converter1/LConn1 -- Ideal Rotational Motion Sensor1/RConn3

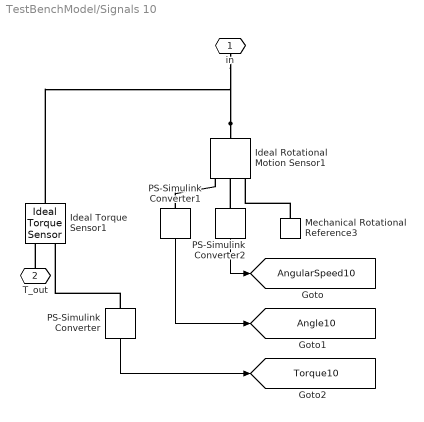
== system TestBenchModel/Signals 10 ==
  Ideal Rotational Motion Sensor1 : fl_lib/Mechanical/Mechanical Sensors/Ideal Rotational Motion Sensor  offset=0 rad
  Ideal Torque Sensor1 : fl_lib/Mechanical/Mechanical Sensors/Ideal Torque Sensor
  Mechanical Rotational Reference3 : fl_lib/Mechanical/Rotational Elements/Mechanical Rotational Reference
  PS-Simulink Converter : nesl_utility/PS-Simulink Converter  PhysicalDomain=network_engine_domain  SubClassName=ps_output  LeftPortType=input  RightPortType=output  PseudoPeriodic=off  Frequencies=[]  Unit=N*m  AffineConversion=off
  PS-Simulink Converter1 : nesl_utility/PS-Simulink Converter  PhysicalDomain=network_engine_domain  SubClassName=ps_output  LeftPortType=input  RightPortType=output  PseudoPeriodic=off  Frequencies=[]  Unit=1  AffineConversion=off
  PS-Simulink Converter2 : nesl_utility/PS-Simulink Converter  PhysicalDomain=network_engine_domain  SubClassName=ps_output  LeftPortType=input  RightPortType=output  PseudoPeriodic=off  Frequencies=[]  Unit=1  AffineConversion=off
  in : PMIOPort  Side=Left
  T_out : PMIOPort  Port=2  Side=Right
  tag scope: Angle10=global, AngularSpeed10=global, Torque10=global
  wires:
  PS-Simulink Converter/1 -> [Torque10]
  PS-Simulink Converter1/1 -> [Angle10]
  PS-Simulink Converter2/1 -> [AngularSpeed10]
  connections:
  PS-Simulink Converter/LConn1 -- Ideal Torque Sensor1/RConn2
  T_out/RConn1 -- Ideal Torque Sensor1/RConn1
  Mechanical Rotational Reference3/LConn1 -- Ideal Rotational Motion Sensor1/RConn1
  PS-Simulink Converter2/LConn1 -- Ideal Rotational Motion Sensor1/RConn2
  Ideal Rotational Motion Sensor1/LConn1 -- Ideal Torque Sensor1/LConn1 -- in/RConn1
  PS-Simulink Converter1/LConn1 -- Ideal Rotational Motion Sensor1/RConn3

== system TestBenchModel/Signals 11 ==
  Ideal Rotational Motion Sensor1 : fl_lib/Mechanical/Mechanical Sensors/Ideal Rotational Motion Sensor  offset=0 rad
  Ideal Torque Sensor1 : fl_lib/Mechanical/Mechanical Sensors/Ideal Torque Sensor
  Mechanical Rotational Reference3 : fl_lib/Mechanical/Rotational Elements/Mechanical Rotational Reference
  PS-Simulink Converter : nesl_utility/PS-Simulink Converter  PhysicalDomain=network_engine_domain  SubClassName=ps_output  LeftPortType=input  RightPortType=output  PseudoPeriodic=off  Frequencies=[]  Unit=N*m  AffineConversion=off
  PS-Simulink Converter1 : nesl_utility/PS-Simulink Converter  PhysicalDomain=network_engine_domain  SubClassName=ps_output  LeftPortType=input  RightPortType=output  PseudoPeriodic=off  Frequencies=[]  Unit=1  AffineConversion=off
  PS-Simulink Converter2 : nesl_utility/PS-Simulink Converter  PhysicalDomain=network_engine_domain  SubClassName=ps_output  LeftPortType=input  RightPortType=output  PseudoPeriodic=off  Frequencies=[]  Unit=1  AffineConversion=off
  in : PMIOPort  Side=Left
  T_out : PMIOPort  Port=2  Side=Right
  tag scope: Angle11=global, AngularSpeed11=global, Torque11=global
  wires:
  PS-Simulink Converter2/1 -> [AngularSpeed11]
  PS-Simulink Converter1/1 -> [Angle11]
  PS-Simulink Converter/1 -> [Torque11]
  connections:
  PS-Simulink Converter1/LConn1 -- Ideal Rotational Motion Sensor1/RConn3
  in/RConn1 -- Ideal Torque Sensor1/LConn1 -- Ideal Rotational Motion Sensor1/LConn1
  PS-Simulink Converter2/LConn1 -- Ideal Rotational Motion Sensor1/RConn2
  Mechanical Rotational Reference3/LConn1 -- Ideal Rotational Motion Sensor1/RConn1
  T_out/RConn1 -- Ideal Torque Sensor1/RConn1
  PS-Simulink Converter/LConn1 -- Ideal Torque Sensor1/RConn2

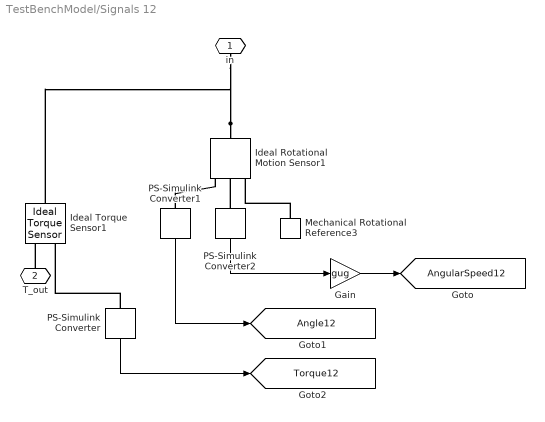
== system TestBenchModel/Signals 12 ==
  Gain : Gain  Gain=gug
  Ideal Rotational Motion Sensor1 : fl_lib/Mechanical/Mechanical Sensors/Ideal Rotational Motion Sensor  offset=0 rad
  Ideal Torque Sensor1 : fl_lib/Mechanical/Mechanical Sensors/Ideal Torque Sensor
  Mechanical Rotational Reference3 : fl_lib/Mechanical/Rotational Elements/Mechanical Rotational Reference
  PS-Simulink Converter : nesl_utility/PS-Simulink Converter  PhysicalDomain=network_engine_domain  SubClassName=ps_output  LeftPortType=input  RightPortType=output  PseudoPeriodic=off  Frequencies=[]  Unit=N*m  AffineConversion=off
  PS-Simulink Converter1 : nesl_utility/PS-Simulink Converter  PhysicalDomain=network_engine_domain  SubClassName=ps_output  LeftPortType=input  RightPortType=output  PseudoPeriodic=off  Frequencies=[]  Unit=1  AffineConversion=off
  PS-Simulink Converter2 : nesl_utility/PS-Simulink Converter  PhysicalDomain=network_engine_domain  SubClassName=ps_output  LeftPortType=input  RightPortType=output  PseudoPeriodic=off  Frequencies=[]  Unit=1  AffineConversion=off
  in : PMIOPort  Side=Left
  T_out : PMIOPort  Port=2  Side=Right
  tag scope: Angle12=global, AngularSpeed12=global, Torque12=global
  wires:
  Gain/1 -> [AngularSpeed12]
  PS-Simulink Converter2/1 -> Gain/1
  PS-Simulink Converter1/1 -> [Angle12]
  PS-Simulink Converter/1 -> [Torque12]
  connections:
  PS-Simulink Converter1/LConn1 -- Ideal Rotational Motion Sensor1/RConn3
  Ideal Rotational Motion Sensor1/LConn1 -- in/RConn1 -- Ideal Torque Sensor1/LConn1
  PS-Simulink Converter2/LConn1 -- Ideal Rotational Motion Sensor1/RConn2
  Mechanical Rotational Reference3/LConn1 -- Ideal Rotational Motion Sensor1/RConn1
  T_out/RConn1 -- Ideal Torque Sensor1/RConn1
  PS-Simulink Converter/LConn1 -- Ideal Torque Sensor1/RConn2

== system TestBenchModel/Signals 13 ==
  Ideal Rotational Motion Sensor1 : fl_lib/Mechanical/Mechanical Sensors/Ideal Rotational Motion Sensor  offset=0 rad
  Ideal Torque Sensor1 : fl_lib/Mechanical/Mechanical Sensors/Ideal Torque Sensor
  Mechanical Rotational Reference3 : fl_lib/Mechanical/Rotational Elements/Mechanical Rotational Reference
  PS-Simulink Converter : nesl_utility/PS-Simulink Converter  PhysicalDomain=network_engine_domain  SubClassName=ps_output  LeftPortType=input  RightPortType=output  PseudoPeriodic=off  Frequencies=[]  Unit=N*m  AffineConversion=off
  PS-Simulink Converter1 : nesl_utility/PS-Simulink Converter  PhysicalDomain=network_engine_domain  SubClassName=ps_output  LeftPortType=input  RightPortType=output  PseudoPeriodic=off  Frequencies=[]  Unit=1  AffineConversion=off
  PS-Simulink Converter2 : nesl_utility/PS-Simulink Converter  PhysicalDomain=network_engine_domain  SubClassName=ps_output  LeftPortType=input  RightPortType=output  PseudoPeriodic=off  Frequencies=[]  Unit=1  AffineConversion=off
  in : PMIOPort  Side=Left
  T_out : PMIOPort  Port=2  Side=Right
  tag scope: Angle13=global, AngularSpeed13=global, Torque13=global
  wires:
  PS-Simulink Converter/1 -> [Torque13]
  PS-Simulink Converter1/1 -> [Angle13]
  PS-Simulink Converter2/1 -> [AngularSpeed13]
  connections:
  PS-Simulink Converter/LConn1 -- Ideal Torque Sensor1/RConn2
  T_out/RConn1 -- Ideal Torque Sensor1/RConn1
  Mechanical Rotational Reference3/LConn1 -- Ideal Rotational Motion Sensor1/RConn1
  PS-Simulink Converter2/LConn1 -- Ideal Rotational Motion Sensor1/RConn2
  Ideal Rotational Motion Sensor1/LConn1 -- Ideal Torque Sensor1/LConn1 -- in/RConn1
  PS-Simulink Converter1/LConn1 -- Ideal Rotational Motion Sensor1/RConn3

== system TestBenchModel/Signals 14 ==
  Ideal Rotational Motion Sensor1 : fl_lib/Mechanical/Mechanical Sensors/Ideal Rotational Motion Sensor  offset=0 rad
  Ideal Torque Sensor1 : fl_lib/Mechanical/Mechanical Sensors/Ideal Torque Sensor
  Mechanical Rotational Reference3 : fl_lib/Mechanical/Rotational Elements/Mechanical Rotational Reference
  PS-Simulink Converter : nesl_utility/PS-Simulink Converter  PhysicalDomain=network_engine_domain  SubClassName=ps_output  LeftPortType=input  RightPortType=output  PseudoPeriodic=off  Frequencies=[]  Unit=N*m  AffineConversion=off
  PS-Simulink Converter1 : nesl_utility/PS-Simulink Converter  PhysicalDomain=network_engine_domain  SubClassName=ps_output  LeftPortType=input  RightPortType=output  PseudoPeriodic=off  Frequencies=[]  Unit=1  AffineConversion=off
  PS-Simulink Converter2 : nesl_utility/PS-Simulink Converter  PhysicalDomain=network_engine_domain  SubClassName=ps_output  LeftPortType=input  RightPortType=output  PseudoPeriodic=off  Frequencies=[]  Unit=1  AffineConversion=off
  in : PMIOPort  Side=Left
  T_out : PMIOPort  Port=2  Side=Right
  tag scope: Angle14=global, AngularSpeed14=global, Torque14=global
  wires:
  PS-Simulink Converter2/1 -> [AngularSpeed14]
  PS-Simulink Converter1/1 -> [Angle14]
  PS-Simulink Converter/1 -> [Torque14]
  connections:
  PS-Simulink Converter1/LConn1 -- Ideal Rotational Motion Sensor1/RConn3
  in/RConn1 -- Ideal Torque Sensor1/LConn1 -- Ideal Rotational Motion Sensor1/LConn1
  PS-Simulink Converter2/LConn1 -- Ideal Rotational Motion Sensor1/RConn2
  Mechanical Rotational Reference3/LConn1 -- Ideal Rotational Motion Sensor1/RConn1
  T_out/RConn1 -- Ideal Torque Sensor1/RConn1
  PS-Simulink Converter/LConn1 -- Ideal Torque Sensor1/RConn2

== system TestBenchModel/Signals 15 ==
  Ideal Rotational Motion Sensor1 : fl_lib/Mechanical/Mechanical Sensors/Ideal Rotational Motion Sensor  offset=0 rad
  Ideal Torque Sensor1 : fl_lib/Mechanical/Mechanical Sensors/Ideal Torque Sensor
  Mechanical Rotational Reference3 : fl_lib/Mechanical/Rotational Elements/Mechanical Rotational Reference
  PS-Simulink Converter : nesl_utility/PS-Simulink Converter  PhysicalDomain=network_engine_domain  SubClassName=ps_output  LeftPortType=input  RightPortType=output  PseudoPeriodic=off  Frequencies=[]  Unit=N*m  AffineConversion=off
  PS-Simulink Converter1 : nesl_utility/PS-Simulink Converter  PhysicalDomain=network_engine_domain  SubClassName=ps_output  LeftPortType=input  RightPortType=output  PseudoPeriodic=off  Frequencies=[]  Unit=1  AffineConversion=off
  PS-Simulink Converter2 : nesl_utility/PS-Simulink Converter  PhysicalDomain=network_engine_domain  SubClassName=ps_output  LeftPortType=input  RightPortType=output  PseudoPeriodic=off  Frequencies=[]  Unit=1  AffineConversion=off
  in : PMIOPort  Side=Left
  T_out : PMIOPort  Port=2  Side=Right
  tag scope: Angle15=global, AngularSpeed15=global, Torque15=global
  wires:
  PS-Simulink Converter/1 -> [Torque15]
  PS-Simulink Converter1/1 -> [Angle15]
  PS-Simulink Converter2/1 -> [AngularSpeed15]
  connections:
  PS-Simulink Converter/LConn1 -- Ideal Torque Sensor1/RConn2
  T_out/RConn1 -- Ideal Torque Sensor1/RConn1
  Mechanical Rotational Reference3/LConn1 -- Ideal Rotational Motion Sensor1/RConn1
  PS-Simulink Converter2/LConn1 -- Ideal Rotational Motion Sensor1/RConn2
  Ideal Rotational Motion Sensor1/LConn1 -- Ideal Torque Sensor1/LConn1 -- in/RConn1
  PS-Simulink Converter1/LConn1 -- Ideal Rotational Motion Sensor1/RConn3

== system TestBenchModel/Signals 16 ==
  Ideal Rotational Motion Sensor1 : fl_lib/Mechanical/Mechanical Sensors/Ideal Rotational Motion Sensor  offset=0 rad
  Ideal Torque Sensor1 : fl_lib/Mechanical/Mechanical Sensors/Ideal Torque Sensor
  Mechanical Rotational Reference3 : fl_lib/Mechanical/Rotational Elements/Mechanical Rotational Reference
  PS-Simulink Converter : nesl_utility/PS-Simulink Converter  PhysicalDomain=network_engine_domain  SubClassName=ps_output  LeftPortType=input  RightPortType=output  PseudoPeriodic=off  Frequencies=[]  Unit=N*m  AffineConversion=off
  PS-Simulink Converter1 : nesl_utility/PS-Simulink Converter  PhysicalDomain=network_engine_domain  SubClassName=ps_output  LeftPortType=input  RightPortType=output  PseudoPeriodic=off  Frequencies=[]  Unit=1  AffineConversion=off
  PS-Simulink Converter2 : nesl_utility/PS-Simulink Converter  PhysicalDomain=network_engine_domain  SubClassName=ps_output  LeftPortType=input  RightPortType=output  PseudoPeriodic=off  Frequencies=[]  Unit=1  AffineConversion=off
  in : PMIOPort  Side=Left
  T_out : PMIOPort  Port=2  Side=Right
  tag scope: Angle16=global, AngularSpeed16=global, Torque16=global
  wires:
  PS-Simulink Converter2/1 -> [AngularSpeed16]
  PS-Simulink Converter1/1 -> [Angle16]
  PS-Simulink Converter/1 -> [Torque16]
  connections:
  PS-Simulink Converter1/LConn1 -- Ideal Rotational Motion Sensor1/RConn3
  in/RConn1 -- Ideal Torque Sensor1/LConn1 -- Ideal Rotational Motion Sensor1/LConn1
  PS-Simulink Converter2/LConn1 -- Ideal Rotational Motion Sensor1/RConn2
  Mechanical Rotational Reference3/LConn1 -- Ideal Rotational Motion Sensor1/RConn1
  T_out/RConn1 -- Ideal Torque Sensor1/RConn1
  PS-Simulink Converter/LConn1 -- Ideal Torque Sensor1/RConn2

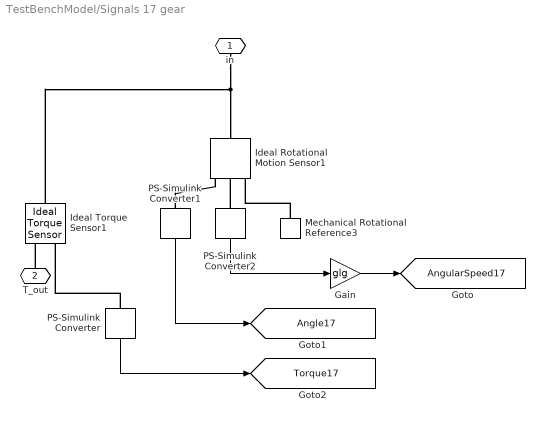
== system TestBenchModel/Signals 17 gear ==
  Gain : Gain  Gain=glg
  Ideal Rotational Motion Sensor1 : fl_lib/Mechanical/Mechanical Sensors/Ideal Rotational Motion Sensor  offset=0 rad
  Ideal Torque Sensor1 : fl_lib/Mechanical/Mechanical Sensors/Ideal Torque Sensor
  Mechanical Rotational Reference3 : fl_lib/Mechanical/Rotational Elements/Mechanical Rotational Reference
  PS-Simulink Converter : nesl_utility/PS-Simulink Converter  PhysicalDomain=network_engine_domain  SubClassName=ps_output  LeftPortType=input  RightPortType=output  PseudoPeriodic=off  Frequencies=[]  Unit=N*m  AffineConversion=off
  PS-Simulink Converter1 : nesl_utility/PS-Simulink Converter  PhysicalDomain=network_engine_domain  SubClassName=ps_output  LeftPortType=input  RightPortType=output  PseudoPeriodic=off  Frequencies=[]  Unit=1  AffineConversion=off
  PS-Simulink Converter2 : nesl_utility/PS-Simulink Converter  PhysicalDomain=network_engine_domain  SubClassName=ps_output  LeftPortType=input  RightPortType=output  PseudoPeriodic=off  Frequencies=[]  Unit=1  AffineConversion=off
  in : PMIOPort  Side=Left
  T_out : PMIOPort  Port=2  Side=Right
  tag scope: Angle17=global, AngularSpeed17=global, Torque17=global
  wires:
  PS-Simulink Converter/1 -> [Torque17]
  PS-Simulink Converter1/1 -> [Angle17]
  PS-Simulink Converter2/1 -> Gain/1
  Gain/1 -> [AngularSpeed17]
  connections:
  PS-Simulink Converter/LConn1 -- Ideal Torque Sensor1/RConn2
  T_out/RConn1 -- Ideal Torque Sensor1/RConn1
  Mechanical Rotational Reference3/LConn1 -- Ideal Rotational Motion Sensor1/RConn1
  PS-Simulink Converter2/LConn1 -- Ideal Rotational Motion Sensor1/RConn2
  Ideal Torque Sensor1/LConn1 -- in/RConn1 -- Ideal Rotational Motion Sensor1/LConn1
  PS-Simulink Converter1/LConn1 -- Ideal Rotational Motion Sensor1/RConn3

== system TestBenchModel/Signals 18 ==
  Ideal Rotational Motion Sensor1 : fl_lib/Mechanical/Mechanical Sensors/Ideal Rotational Motion Sensor  offset=0 rad
  Ideal Torque Sensor1 : fl_lib/Mechanical/Mechanical Sensors/Ideal Torque Sensor
  Mechanical Rotational Reference3 : fl_lib/Mechanical/Rotational Elements/Mechanical Rotational Reference
  PS-Simulink Converter : nesl_utility/PS-Simulink Converter  PhysicalDomain=network_engine_domain  SubClassName=ps_output  LeftPortType=input  RightPortType=output  PseudoPeriodic=off  Frequencies=[]  Unit=N*m  AffineConversion=off
  PS-Simulink Converter1 : nesl_utility/PS-Simulink Converter  PhysicalDomain=network_engine_domain  SubClassName=ps_output  LeftPortType=input  RightPortType=output  PseudoPeriodic=off  Frequencies=[]  Unit=1  AffineConversion=off
  PS-Simulink Converter2 : nesl_utility/PS-Simulink Converter  PhysicalDomain=network_engine_domain  SubClassName=ps_output  LeftPortType=input  RightPortType=output  PseudoPeriodic=off  Frequencies=[]  Unit=1  AffineConversion=off
  in : PMIOPort  Side=Left
  T_out : PMIOPort  Port=2  Side=Right
  tag scope: Angle18=global, AngularSpeed18=global, Torque18=global
  wires:
  PS-Simulink Converter/1 -> [Torque18]
  PS-Simulink Converter1/1 -> [Angle18]
  PS-Simulink Converter2/1 -> [AngularSpeed18]
  connections:
  PS-Simulink Converter/LConn1 -- Ideal Torque Sensor1/RConn2
  T_out/RConn1 -- Ideal Torque Sensor1/RConn1
  Mechanical Rotational Reference3/LConn1 -- Ideal Rotational Motion Sensor1/RConn1
  PS-Simulink Converter2/LConn1 -- Ideal Rotational Motion Sensor1/RConn2
  Ideal Rotational Motion Sensor1/LConn1 -- Ideal Torque Sensor1/LConn1 -- in/RConn1
  PS-Simulink Converter1/LConn1 -- Ideal Rotational Motion Sensor1/RConn3

== system TestBenchModel/Signals 19 ==
  Ideal Rotational Motion Sensor1 : fl_lib/Mechanical/Mechanical Sensors/Ideal Rotational Motion Sensor  offset=0 rad
  Ideal Torque Sensor1 : fl_lib/Mechanical/Mechanical Sensors/Ideal Torque Sensor
  Mechanical Rotational Reference3 : fl_lib/Mechanical/Rotational Elements/Mechanical Rotational Reference
  PS-Simulink Converter : nesl_utility/PS-Simulink Converter  PhysicalDomain=network_engine_domain  SubClassName=ps_output  LeftPortType=input  RightPortType=output  PseudoPeriodic=off  Frequencies=[]  Unit=N*m  AffineConversion=off
  PS-Simulink Converter1 : nesl_utility/PS-Simulink Converter  PhysicalDomain=network_engine_domain  SubClassName=ps_output  LeftPortType=input  RightPortType=output  PseudoPeriodic=off  Frequencies=[]  Unit=1  AffineConversion=off
  PS-Simulink Converter2 : nesl_utility/PS-Simulink Converter  PhysicalDomain=network_engine_domain  SubClassName=ps_output  LeftPortType=input  RightPortType=output  PseudoPeriodic=off  Frequencies=[]  Unit=1  AffineConversion=off
  in : PMIOPort  Side=Left
  T_out : PMIOPort  Port=2  Side=Right
  tag scope: Angle19=global, AngularSpeed19=global, Torque19=global
  wires:
  PS-Simulink Converter2/1 -> [AngularSpeed19]
  PS-Simulink Converter1/1 -> [Angle19]
  PS-Simulink Converter/1 -> [Torque19]
  connections:
  PS-Simulink Converter1/LConn1 -- Ideal Rotational Motion Sensor1/RConn3
  in/RConn1 -- Ideal Torque Sensor1/LConn1 -- Ideal Rotational Motion Sensor1/LConn1
  PS-Simulink Converter2/LConn1 -- Ideal Rotational Motion Sensor1/RConn2
  Mechanical Rotational Reference3/LConn1 -- Ideal Rotational Motion Sensor1/RConn1
  T_out/RConn1 -- Ideal Torque Sensor1/RConn1
  PS-Simulink Converter/LConn1 -- Ideal Torque Sensor1/RConn2

== system TestBenchModel/Signals 2 ==
  Ideal Rotational Motion Sensor1 : fl_lib/Mechanical/Mechanical Sensors/Ideal Rotational Motion Sensor  offset=0 rad
  Ideal Torque Sensor1 : fl_lib/Mechanical/Mechanical Sensors/Ideal Torque Sensor
  Mechanical Rotational Reference3 : fl_lib/Mechanical/Rotational Elements/Mechanical Rotational Reference
  PS-Simulink Converter : nesl_utility/PS-Simulink Converter  PhysicalDomain=network_engine_domain  SubClassName=ps_output  LeftPortType=input  RightPortType=output  PseudoPeriodic=off  Frequencies=[]  Unit=N*m  AffineConversion=off
  PS-Simulink Converter1 : nesl_utility/PS-Simulink Converter  PhysicalDomain=network_engine_domain  SubClassName=ps_output  LeftPortType=input  RightPortType=output  PseudoPeriodic=off  Frequencies=[]  Unit=1  AffineConversion=off
  PS-Simulink Converter2 : nesl_utility/PS-Simulink Converter  PhysicalDomain=network_engine_domain  SubClassName=ps_output  LeftPortType=input  RightPortType=output  PseudoPeriodic=off  Frequencies=[]  Unit=1  AffineConversion=off
  in : PMIOPort  Side=Left
  T_out : PMIOPort  Port=2  Side=Right
  tag scope: Angle2=global, AngularSpeed2=global, Torque2=global
  wires:
  PS-Simulink Converter2/1 -> [AngularSpeed2]
  PS-Simulink Converter1/1 -> [Angle2]
  PS-Simulink Converter/1 -> [Torque2]
  connections:
  PS-Simulink Converter1/LConn1 -- Ideal Rotational Motion Sensor1/RConn3
  in/RConn1 -- Ideal Torque Sensor1/LConn1 -- Ideal Rotational Motion Sensor1/LConn1
  PS-Simulink Converter2/LConn1 -- Ideal Rotational Motion Sensor1/RConn2
  Mechanical Rotational Reference3/LConn1 -- Ideal Rotational Motion Sensor1/RConn1
  T_out/RConn1 -- Ideal Torque Sensor1/RConn1
  PS-Simulink Converter/LConn1 -- Ideal Torque Sensor1/RConn2

== system TestBenchModel/Signals 20 ==
  Ideal Rotational Motion Sensor1 : fl_lib/Mechanical/Mechanical Sensors/Ideal Rotational Motion Sensor  offset=0 rad
  Ideal Torque Sensor1 : fl_lib/Mechanical/Mechanical Sensors/Ideal Torque Sensor
  Mechanical Rotational Reference3 : fl_lib/Mechanical/Rotational Elements/Mechanical Rotational Reference
  PS-Simulink Converter : nesl_utility/PS-Simulink Converter  PhysicalDomain=network_engine_domain  SubClassName=ps_output  LeftPortType=input  RightPortType=output  PseudoPeriodic=off  Frequencies=[]  Unit=N*m  AffineConversion=off
  PS-Simulink Converter1 : nesl_utility/PS-Simulink Converter  PhysicalDomain=network_engine_domain  SubClassName=ps_output  LeftPortType=input  RightPortType=output  PseudoPeriodic=off  Frequencies=[]  Unit=1  AffineConversion=off
  PS-Simulink Converter2 : nesl_utility/PS-Simulink Converter  PhysicalDomain=network_engine_domain  SubClassName=ps_output  LeftPortType=input  RightPortType=output  PseudoPeriodic=off  Frequencies=[]  Unit=1  AffineConversion=off
  in : PMIOPort  Side=Left
  T_out : PMIOPort  Port=2  Side=Right
  tag scope: Angle20=global, AngularSpeed20=global, Torque20=global
  wires:
  PS-Simulink Converter/1 -> [Torque20]
  PS-Simulink Converter1/1 -> [Angle20]
  PS-Simulink Converter2/1 -> [AngularSpeed20]
  connections:
  PS-Simulink Converter/LConn1 -- Ideal Torque Sensor1/RConn2
  T_out/RConn1 -- Ideal Torque Sensor1/RConn1
  Mechanical Rotational Reference3/LConn1 -- Ideal Rotational Motion Sensor1/RConn1
  PS-Simulink Converter2/LConn1 -- Ideal Rotational Motion Sensor1/RConn2
  Ideal Rotational Motion Sensor1/LConn1 -- Ideal Torque Sensor1/LConn1 -- in/RConn1
  PS-Simulink Converter1/LConn1 -- Ideal Rotational Motion Sensor1/RConn3
